simulink model "modele_corde"  (R2019b)
settings: Solver=VariableStepAuto  StartTime=0.0  StopTime=10  MaxStep=0.1  RelTol=1e-3
libraries: simulink x1
settings Model: Creator=eric  LastModifiedBy=jeanz
settings DataIOCC: ReturnWorkspaceOutputs=off
settings DebuggingCC: ArithmeticOperatorsInVariantConditions=warning
settings SFSimCC: SimUseLocalCustomCode=off  CustomCodeUndefinedFunction=UseInterfaceOnly
settings RTWCC: RTWUseLocalCustomCode=off

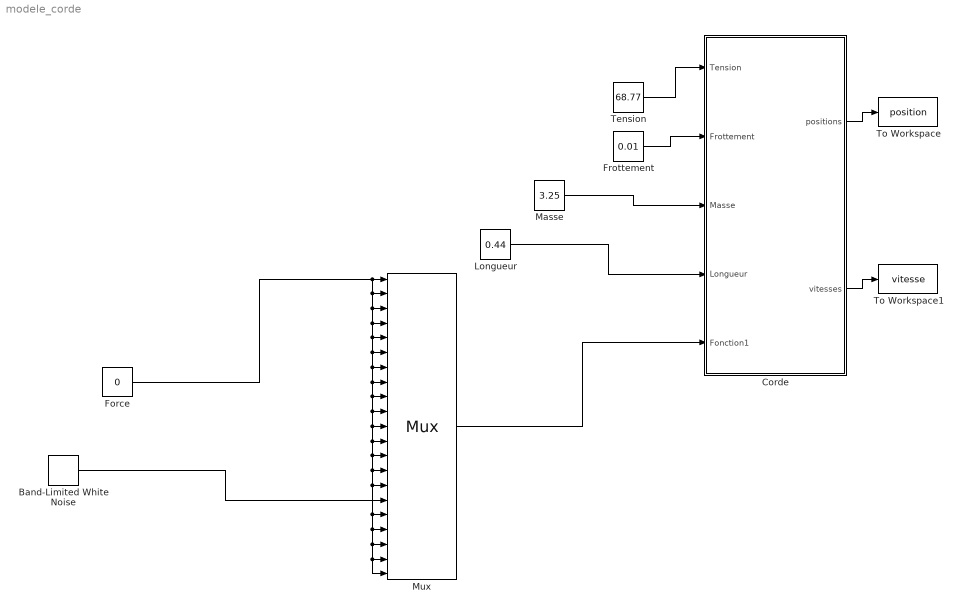
== system modele_corde ==
  Band-Limited White Noise : simulink/Sources/Band-Limited White Noise  Cov=[0.1]  Ts=0.1  seed=[23341]
  Corde : Subsystem
  Force : Constant  Value=0
  Frottement : Constant  Value=0.01
  Longueur : Constant  Value=0.44
  Masse : Constant  Value=3.25
  Mux : Mux  Inputs=21
  Tension : Constant  Value=68.77
  To Workspace : ToWorkspace  VariableName=position  SaveFormat=Timeseries  SampleTime=0.05
  To Workspace1 : ToWorkspace  VariableName=vitesse  SaveFormat=Timeseries  SampleTime=0.05
  wires:
  Tension/1 -> Corde/1(Tension)
  Frottement/1 -> Corde/2(Frottement)
  Masse/1 -> Corde/3(Masse)
  Longueur/1 -> Corde/4(Longueur)
  Corde/1(positions) -> To Workspace/1
  Corde/2(vitesses) -> To Workspace1/1
  Mux/1 -> Corde/5(Fonction1)
  Force/1 -> Mux/6, Mux/11, Mux/12, Mux/21, Mux/20, Mux/19, Mux/18, Mux/17, Mux/15, Mux/14, Mux/13, Mux/10, Mux/9, Mux/8, Mux/7, Mux/5, Mux/4, Mux/3, Mux/2, Mux/1
  Band-Limited White Noise/1 -> Mux/16

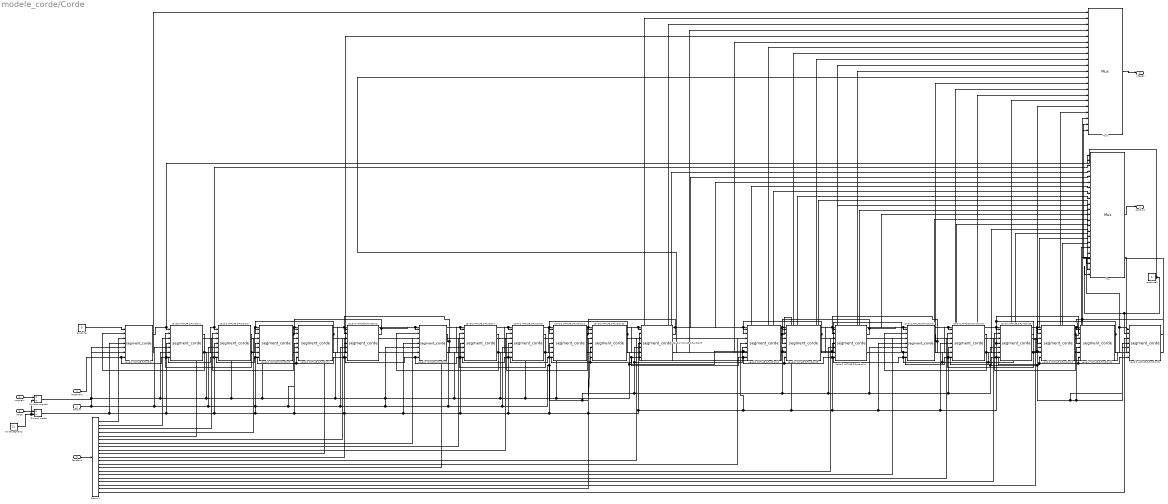
== system modele_corde/Corde ==
  Tension : Inport
  Frottement : Inport  Port=2
  Masse : Inport  Port=3
  Longueur : Inport  Port=4
  Fonction1 : Inport  Port=5
  Demux1 : Demux  Outputs=21
  Division longueur : Product  Inputs=*/
  Division masse : Product  Inputs=*/
  Level-2 MATLAB S-Function{,1..20} (21 alike) : M-S-Function  FunctionName=segment_corde
  Mux : Mux  Inputs=23
  Mux1 : Mux  Inputs=21
  extrémité : Constant  Value=0
  extrémité1 : Constant  Value=0
  nbr de segments : Constant  Value=21
  positions : Outport  VectorParamsAs1DForOutWhenUnconnected=off
  vitesses : Outport  Port=2  VectorParamsAs1DForOutWhenUnconnected=off
  wires:
  Level-2 MATLAB S-Function4/1 -> Level-2 MATLAB S-Function5/2, Level-2 MATLAB S-Function3/1, Mux/6
  Level-2 MATLAB S-Function1/1 -> Level-2 MATLAB S-Function/2, Mux/3, Level-2 MATLAB S-Function2/1
  Level-2 MATLAB S-Function5/1 -> Mux/5, Level-2 MATLAB S-Function4/1, Level-2 MATLAB S-Function2/2
  Level-2 MATLAB S-Function2/1 -> Level-2 MATLAB S-Function1/2, Mux/4, Level-2 MATLAB S-Function5/1
  Level-2 MATLAB S-Function3/1 -> Level-2 MATLAB S-Function6/1, Mux/7, Level-2 MATLAB S-Function4/2
  extrémité/1 -> Level-2 MATLAB S-Function/1
  Level-2 MATLAB S-Function7/1 -> Level-2 MATLAB S-Function6/2, Level-2 MATLAB S-Function8/1, Mux/9
  Level-2 MATLAB S-Function9/1 -> Level-2 MATLAB S-Function16/1, Mux/13, Level-2 MATLAB S-Function10/2
  Level-2 MATLAB S-Function8/1 -> Level-2 MATLAB S-Function7/2, Level-2 MATLAB S-Function11/1, Mux/10
  Level-2 MATLAB S-Function11/1 -> Level-2 MATLAB S-Function10/1, Mux/11, Level-2 MATLAB S-Function8/2
  Level-2 MATLAB S-Function6/1 -> Level-2 MATLAB S-Function7/1, Mux/8, Level-2 MATLAB S-Function3/2
  Level-2 MATLAB S-Function10/1 -> Level-2 MATLAB S-Function11/2, Mux/12, Level-2 MATLAB S-Function9/1
  Division masse/1 -> Level-2 MATLAB S-Function1/4, Level-2 MATLAB S-Function2/4, Level-2 MATLAB S-Function5/4, Level-2 MATLAB S-Function4/4, Level-2 MATLAB S-Function7/4, Level-2 MATLAB S-Function8/4, Level-2 MATLAB S-Function11/4, Level-2 MATLAB S-Function10/4, Level-2 MATLAB S-Function16/4, Level-2 MATLAB S-Function12/4, Level-2 MATLAB S-Function13/4, Level-2 MATLAB S-Function19/4, Level-2 MATLAB S-Function18/4, Level-2 MATLAB S-Function17/4, Level-2 MATLAB S-Function14/4, Level-2 MATLAB S-Function15/4, Level-2 MATLAB S-Function9/4, Level-2 MATLAB S-Function6/4, Level-2 MATLAB S-Function3/4, Level-2 MATLAB S-Function/4
  Level-2 MATLAB S-Function16/1 -> Level-2 MATLAB S-Function15/1, Mux/14, Level-2 MATLAB S-Function9/2
  Tension/1 -> Level-2 MATLAB S-Function2/5, Level-2 MATLAB S-Function5/5, Level-2 MATLAB S-Function4/5, Level-2 MATLAB S-Function3/5, Level-2 MATLAB S-Function8/5, Level-2 MATLAB S-Function11/5, Level-2 MATLAB S-Function13/5, Level-2 MATLAB S-Function20/5, Level-2 MATLAB S-Function20/4, Level-2 MATLAB S-Function12/5, Level-2 MATLAB S-Function19/5, Level-2 MATLAB S-Function18/5, Level-2 MATLAB S-Function17/5, Level-2 MATLAB S-Function14/5, Level-2 MATLAB S-Function15/5, Level-2 MATLAB S-Function9/5, Level-2 MATLAB S-Function16/5, Level-2 MATLAB S-Function10/5, Level-2 MATLAB S-Function7/5, Level-2 MATLAB S-Function6/5, Level-2 MATLAB S-Function1/5, Level-2 MATLAB S-Function/5
  Division longueur/1 -> Level-2 MATLAB S-Function9/6, Level-2 MATLAB S-Function20/6, Level-2 MATLAB S-Function12/6, Level-2 MATLAB S-Function13/6, Level-2 MATLAB S-Function19/6, Level-2 MATLAB S-Function18/6, Level-2 MATLAB S-Function17/6, Level-2 MATLAB S-Function14/6, Level-2 MATLAB S-Function15/6, Level-2 MATLAB S-Function16/6, Level-2 MATLAB S-Function10/6, Level-2 MATLAB S-Function11/6, Level-2 MATLAB S-Function8/6, Level-2 MATLAB S-Function7/6, Level-2 MATLAB S-Function6/6, Level-2 MATLAB S-Function3/6, Level-2 MATLAB S-Function4/6, Level-2 MATLAB S-Function5/6, Level-2 MATLAB S-Function2/6, Level-2 MATLAB S-Function1/6, Level-2 MATLAB S-Function/6
  Level-2 MATLAB S-Function20/1 -> Level-2 MATLAB S-Function12/2, Mux/22
  Level-2 MATLAB S-Function14/1 -> Level-2 MATLAB S-Function17/1, Mux/16, Level-2 MATLAB S-Function15/2
  Level-2 MATLAB S-Function19/1 -> Level-2 MATLAB S-Function18/2, Level-2 MATLAB S-Function13/1, Mux/19
  Level-2 MATLAB S-Function15/1 -> Level-2 MATLAB S-Function16/2, Level-2 MATLAB S-Function14/1, Mux/15
  Level-2 MATLAB S-Function13/1 -> Level-2 MATLAB S-Function12/1, Mux/20, Level-2 MATLAB S-Function19/2
  Level-2 MATLAB S-Function17/1 -> Level-2 MATLAB S-Function18/1, Mux/17, Level-2 MATLAB S-Function14/2
  Level-2 MATLAB S-Function18/1 -> Level-2 MATLAB S-Function17/2, Level-2 MATLAB S-Function19/1, Mux/18
  Level-2 MATLAB S-Function12/1 -> Level-2 MATLAB S-Function13/2, Mux/21, Level-2 MATLAB S-Function20/1
  extrémité1/1 -> Mux/1, Mux/23, Level-2 MATLAB S-Function20/2
  Mux/1 -> positions/1
  Mux1/1 -> vitesses/1
  Level-2 MATLAB S-Function1/2 -> Mux1/2
  Level-2 MATLAB S-Function2/2 -> Mux1/3
  Level-2 MATLAB S-Function5/2 -> Mux1/4
  Level-2 MATLAB S-Function4/2 -> Mux1/5
  Level-2 MATLAB S-Function3/2 -> Mux1/6
  Level-2 MATLAB S-Function6/2 -> Mux1/7
  Level-2 MATLAB S-Function7/2 -> Mux1/8
  Level-2 MATLAB S-Function8/2 -> Mux1/9
  Level-2 MATLAB S-Function11/2 -> Mux1/10
  Level-2 MATLAB S-Function10/2 -> Mux1/11
  Level-2 MATLAB S-Function9/2 -> Mux1/12
  Level-2 MATLAB S-Function16/2 -> Mux1/13
  Level-2 MATLAB S-Function15/2 -> Mux1/14
  Level-2 MATLAB S-Function14/2 -> Mux1/15
  Level-2 MATLAB S-Function17/2 -> Mux1/16
  Level-2 MATLAB S-Function18/2 -> Mux1/17
  Level-2 MATLAB S-Function19/2 -> Mux1/18
  Level-2 MATLAB S-Function13/2 -> Mux1/19
  Level-2 MATLAB S-Function12/2 -> Mux1/20
  Level-2 MATLAB S-Function20/2 -> Mux1/21
  Fonction1/1 -> Demux1/1
  nbr de segments/1 -> Division longueur/2, Division masse/2
  Masse/1 -> Division masse/1
  Longueur/1 -> Division longueur/1
  Level-2 MATLAB S-Function/1 -> Mux/2, Level-2 MATLAB S-Function1/1
  Level-2 MATLAB S-Function/2 -> Mux1/1
  Demux1/1 -> Level-2 MATLAB S-Function/3
  Demux1/2 -> Level-2 MATLAB S-Function1/3
  Demux1/3 -> Level-2 MATLAB S-Function2/3
  Demux1/4 -> Level-2 MATLAB S-Function5/3
  Demux1/5 -> Level-2 MATLAB S-Function4/3
  Demux1/6 -> Level-2 MATLAB S-Function3/3
  Demux1/7 -> Level-2 MATLAB S-Function6/3
  Demux1/8 -> Level-2 MATLAB S-Function7/3
  Demux1/9 -> Level-2 MATLAB S-Function8/3
  Demux1/10 -> Level-2 MATLAB S-Function11/3
  Demux1/11 -> Level-2 MATLAB S-Function10/3
  Demux1/12 -> Level-2 MATLAB S-Function9/3
  Demux1/13 -> Level-2 MATLAB S-Function16/3
  Demux1/14 -> Level-2 MATLAB S-Function15/3
  Demux1/15 -> Level-2 MATLAB S-Function14/3
  Demux1/16 -> Level-2 MATLAB S-Function17/3
  Demux1/17 -> Level-2 MATLAB S-Function18/3
  Demux1/18 -> Level-2 MATLAB S-Function19/3
  Demux1/19 -> Level-2 MATLAB S-Function13/3
  Demux1/20 -> Level-2 MATLAB S-Function12/3
  Demux1/21 -> Level-2 MATLAB S-Function20/3
  Frottement/1 -> Level-2 MATLAB S-Function4/7, Level-2 MATLAB S-Function10/7, Level-2 MATLAB S-Function9/7, Level-2 MATLAB S-Function15/7, Level-2 MATLAB S-Function13/7, Level-2 MATLAB S-Function12/7, Level-2 MATLAB S-Function20/7, Level-2 MATLAB S-Function19/7, Level-2 MATLAB S-Function18/7, Level-2 MATLAB S-Function17/7, Level-2 MATLAB S-Function14/7, Level-2 MATLAB S-Function16/7, Level-2 MATLAB S-Function11/7, Level-2 MATLAB S-Function8/7, Level-2 MATLAB S-Function7/7, Level-2 MATLAB S-Function6/7, Level-2 MATLAB S-Function3/7, Level-2 MATLAB S-Function5/7, Level-2 MATLAB S-Function2/7, Level-2 MATLAB S-Function1/7, Level-2 MATLAB S-Function/7
